simulink model "ChevilleNAO_Complete"  (R2015a)
settings: Solver=ode23t  StartTime=0.0  StopTime=2  MaxStep=0.001  RelTol=1e-3
undefined symbols (not defined in the file): X, Y, Z
libraries: sm_lib x306, fl_lib x13, nesl_utility x6
(part 1 of 7)
settings Model: CovSFcnEnable=off  Creator=Xavier  LastModifiedBy=Xavier
settings SolverCC: AlgebraicLoopSolver=LineSearch
settings DebuggingCC: SolverPrmCheckMsg=warning

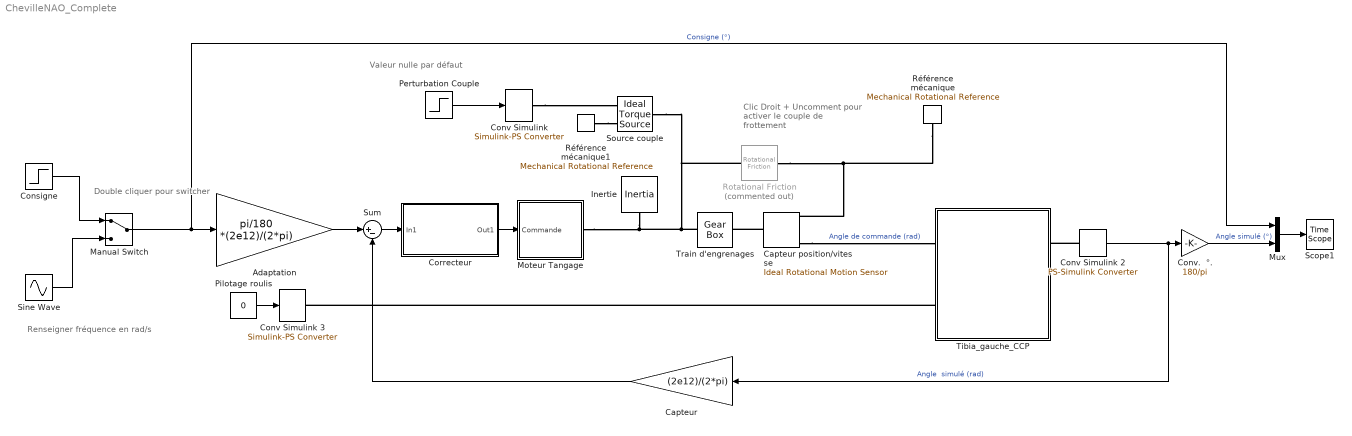
== system ChevilleNAO_Complete ==
  note: Clic Droit + Uncomment pour activer le couple de frottement
  note: Valeur nulle par défaut
  note: Double cliquer pour switcher
  note: Renseigner fréquence en rad/s
  Adaptation : Gain  Gain=pi/180 *(2e12)/(2*pi)
  Capteur : Gain  Gain=(2e12)/(2*pi)
  Capteur position/vitesse : fl_lib/Mechanical/Mechanical Sensors/Ideal Rotational Motion Sensor  offset=0 rad
  Consigne : Step  Time=0  After=5  SampleTime=0
  Conv Simulink 2 : nesl_utility/PS-Simulink Converter  PhysicalDomain=network_engine_domain  SubClassName=ps_output  LeftPortType=input  RightPortType=output  PseudoPeriodic=off  Frequencies=[]  Unit=1  AffineConversion=off
  Conv Simulink 3 : nesl_utility/Simulink-PS Converter  PhysicalDomain=network_engine_domain  SubClassName=ps_input  LeftPortType=input  RightPortType=output  PseudoPeriodic=off  Frequencies=[]  NoiseDistribution=none  NoiseParameters=[]  Unit=1  AffineConversion=off  InputFiltering=off  SimscapeFilterOrder=1  InputFilterTimeConstant=0.001  UdotUserProvided=1
  Conv Simulink : nesl_utility/Simulink-PS Converter  PhysicalDomain=network_engine_domain  SubClassName=ps_input  LeftPortType=input  RightPortType=output  PseudoPeriodic=off  Frequencies=[]  NoiseDistribution=none  NoiseParameters=[]  Unit=1  AffineConversion=off  InputFiltering=off  SimscapeFilterOrder=1  InputFilterTimeConstant=0.001  UdotUserProvided=1
  Conv.  °. : Gain  Gain=180/pi
  Correcteur : Subsystem
      mask Display: image(imread('carte.png'))
  Inertie : fl_lib/Mechanical/Rotational Elements/Inertia  inertia=4.8e-7 kg*m^2  w_specify=off  w_priority=High  w=0 rad/s  t_specify=off  t_priority=High  t=0 N*m
  Manual Switch : ManualSwitch
  Moteur Tangage : Subsystem
      mask Display: image(imread('moteur.png'))
  Mux : Mux  Inputs=2
  Perturbation Couple : Step  Time=0  After=-3.5E-3*0  SampleTime=0
  Pilotage roulis : Constant  Value=0
  Rotational Friction : fl_lib/Mechanical/Rotational Elements/Rotational Friction  Commented=on  brkwy_trq=5 mN*m  Col_trq=5 mN*m  visc_coef=10e-10 N*m/(rad/s)  trans_coef=10 s/rad  vel_thr=1e-4 rad/s  w_specify=off  w_priority=High  w=0 rad/s  t_specify=off  t_priority=High  t=0 N*m
  Référence mécanique : fl_lib/Mechanical/Rotational Elements/Mechanical Rotational Reference
  Référence mécanique1 : fl_lib/Mechanical/Rotational Elements/Mechanical Rotational Reference
  Scope1 : TimeScope
  Sine Wave : Sin  SampleTime=0
  Source couple : fl_lib/Mechanical/Mechanical Sources/Ideal Torque Source
  Sum : Sum  Inputs=|+-
  Tibia_gauche_CCP : Subsystem
      mask Display: image(imread('TibiaCCP.png'))
  Train d'engrenages : fl_lib/Mechanical/Mechanisms/Gear Box  ratio=130.85  t_in_specify=off  t_in_priority=High  t_in=0 N*m  t_out_specify=off  t_out_priority=High  t_out=0 N*m
  wires:
  Pilotage roulis/1 -> Conv Simulink 3/1
  Conv Simulink 2/1 -> Conv.  °./1, Capteur/1  "Angle  simulé (rad)"
  Manual Switch/1 -> Mux/1, Adaptation/1  "Consigne (°)"
  Adaptation/1 -> Sum/1
  Conv.  °./1 -> Mux/2  "Angle simulé (°)"
  Mux/1 -> Scope1/1
  Perturbation Couple/1 -> Conv Simulink/1
  Capteur/1 -> Sum/2
  Sum/1 -> Correcteur/1(In1)
  Correcteur/1(Out1) -> Moteur Tangage/1(Commande)
  Consigne/1 -> Manual Switch/1
  Sine Wave/1 -> Manual Switch/2
  connections:
  Train d'engrenages/LConn1 -- Rotational Friction/LConn1 -- Source couple/LConn1 -- Moteur Tangage/RConn1 -- Inertie/LConn1
  Tibia_gauche_CCP/LConn2 -- Conv Simulink 3/RConn1
  Capteur position/vitesse/LConn1 -- Train d'engrenages/RConn1
  Conv Simulink 2/LConn1 -- Tibia_gauche_CCP/RConn1
  Capteur position/vitesse/RConn3 -- Tibia_gauche_CCP/LConn1  "Angle de commande (rad)"
  Conv Simulink/RConn1 -- Source couple/RConn1
  Référence mécanique1/LConn1 -- Source couple/RConn2
  Référence mécanique/LConn1 -- Rotational Friction/RConn1 -- Capteur position/vitesse/RConn1

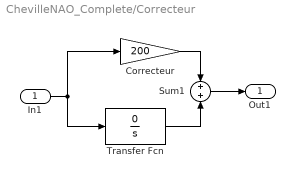
== system ChevilleNAO_Complete/Correcteur ==
  In1 : Inport
  Correcteur : Gain  Gain=200
  Sum1 : Sum
  Transfer Fcn : TransferFcn  Numerator=[0]  Denominator=[1 0]
  Out1 : Outport
  wires:
  In1/1 -> Transfer Fcn/1, Correcteur/1
  Sum1/1 -> Out1/1
  Transfer Fcn/1 -> Sum1/2
  Correcteur/1 -> Sum1/1

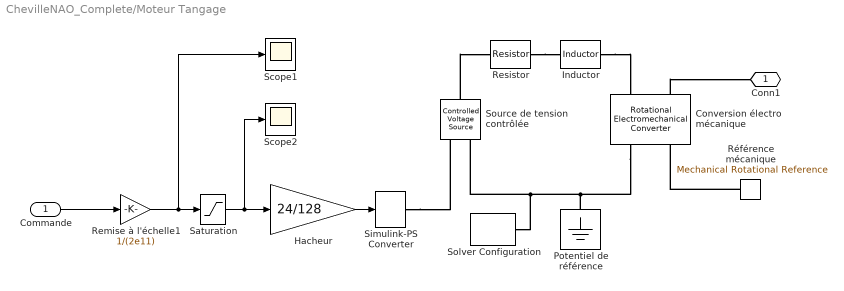
== system ChevilleNAO_Complete/Moteur Tangage ==
  Commande : Inport
  Conversion électro mécanique : fl_lib/Electrical/Electrical Elements/Rotational Electromechanical Converter  K=0.00203 V/rpm  i_specify=off  i_priority=High  i=0 A  v_specify=off  v_priority=High  v=0 V  t_specify=off  t_priority=High  t=0 N*m  w_specify=off  w_priority=High  w=0 rad/s
  Hacheur : Gain  Gain=24/128
  Inductor : fl_lib/Electrical/Electrical Elements/Inductor  l=0.6 mH  r=0 Ohm  g=1e-9 1/Ohm  i_specify=off  i_priority=High  i=0 A  v_specify=off  v_priority=High  v=0 V  i_L_specify=off  i_L_priority=High  i_L=0 A
  Potentiel de référence : fl_lib/Electrical/Electrical Elements/Electrical Reference
  Remise à l'échelle1 : Gain  Gain=1/(2e11)
  Resistor : fl_lib/Electrical/Electrical Elements/Resistor  R=5.4 Ohm  i_specify=off  i_priority=High  i=0 A  v_specify=off  v_priority=High  v=0 V
  Référence mécanique : fl_lib/Mechanical/Rotational Elements/Mechanical Rotational Reference
  Saturation : Saturate  UpperLimit=128  LowerLimit=-128
  Scope1 : Scope
      settings: TimeRange=0.7  YMin=0  YMax=70
  Scope2 : Scope
      settings: TimeRange=1  YMin=0  YMax=60  SaveName=ScopeData3
  Simulink-PS Converter : nesl_utility/Simulink-PS Converter  PhysicalDomain=network_engine_domain  SubClassName=ps_input  LeftPortType=input  RightPortType=output  PseudoPeriodic=off  Frequencies=[]  NoiseDistribution=none  NoiseParameters=[]  Unit=1  AffineConversion=off  InputFiltering=off  SimscapeFilterOrder=1  InputFilterTimeConstant=0.001  UdotUserProvided=1
  Solver Configuration : nesl_utility/Solver Configuration  PhysicalDomain=network_engine_domain  SubClassName=solver  LeftPortType=input  RightPortType=generic  Accelerate=off  Tones=[]  Harmonics=[]  SimulateNoise=off  Profile=off  UseLocalSampling=off  EnableSwitchedLinearOptims=on  FrequencyDomain=off  UseCCode=off  RelTol=0.001  AbsTol=1e-06  MinStep=1e-09  ToWorkspace=off  RevertToSquareIcSolve=off  NumHomotopyIterations=100  DoDC=off  ResidualTolerance=1e-09  UseLocalSolver=off  LocalSolverChoice=NE_BACKWARD_EULER_ADVANCER  LocalSolverSampleTime=0.001  DoFixedCost=off  MaxNonlinIter=3  MaxModeIter=2  LinearAlgebra=Sparse  DelaysMemoryBudget=1024  AutomaticFiltering=on  FilteringTimeConstant=0.001
  Source de tension contrôlée : fl_lib/Electrical/Electrical Sources/Controlled Voltage Source
  Conn1 : PMIOPort  Port=1  Side=Right
  wires:
  Saturation/1 -> Scope2/1, Hacheur/1
  Hacheur/1 -> Simulink-PS Converter/1
  Commande/1 -> Remise à l'échelle1/1
  Remise à l'échelle1/1 -> Scope1/1, Saturation/1
  connections:
  Conversion électro mécanique/LConn2 -- Conn1/RConn1
  Référence mécanique/LConn1 -- Conversion électro mécanique/RConn2
  Source de tension contrôlée/LConn1 -- Resistor/LConn1
  Resistor/RConn1 -- Inductor/LConn1
  Inductor/RConn1 -- Conversion électro mécanique/LConn1
  Conversion électro mécanique/RConn1 -- Potentiel de référence/LConn1 -- Solver Configuration/RConn1 -- Source de tension contrôlée/RConn2
  Simulink-PS Converter/RConn1 -- Source de tension contrôlée/RConn1

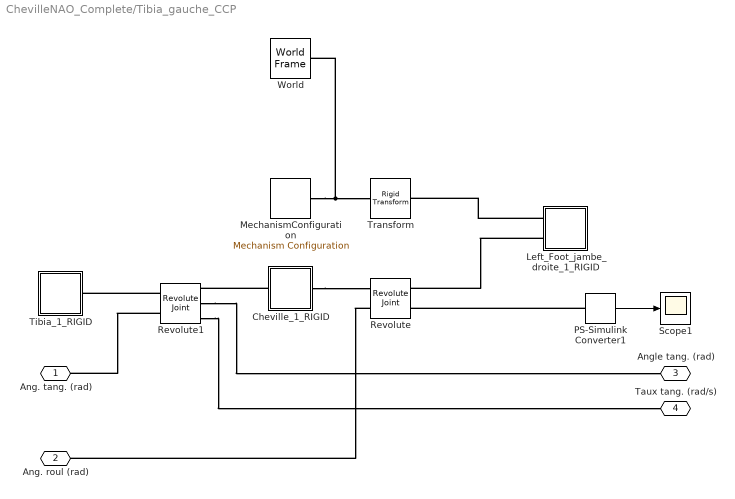
== system ChevilleNAO_Complete/Tibia_gauche_CCP ==
  Cheville_1_RIGID : Subsystem
  Left_Foot_jambe_droite_1_RIGID : Subsystem
  MechanismConfiguration : sm_lib/Utilities/Mechanism Configuration  UniformGravity=Constant  GravityVector=[0 -9.81 0]  GravityUnits=m/s^2  LinearizationDelta=0.001  BlockFunction=simmechanics.library.utilities.mechanism_configuration
  PS-Simulink Converter1 : nesl_utility/PS-Simulink Converter  PhysicalDomain=network_engine_domain  SubClassName=ps_output  LeftPortType=input  RightPortType=output  PseudoPeriodic=off  Frequencies=[]  Unit=1  AffineConversion=off
  Revolute : sm_lib/Joints/Revolute Joint  SenseConstraintForce=off  SenseConstraintForceX=off  SenseConstraintForceY=off  SenseConstraintForceZ=off  SenseConstraintTorque=off  SenseConstraintTorqueX=off  SenseConstraintTorqueY=off  SenseConstraintTorqueZ=off  SenseTotalForce=off  SenseTotalForceX=off  SenseTotalForceY=off  SenseTotalForceZ=off  SenseTotalTorque=off  SenseTotalTorqueX=off  SenseTotalTorqueY=off  SenseTotalTorqueZ=off  CompositeWrenchDir=FollowerOnBase  CompositeWrenchFrame=BaseFrame  EquilibriumPosition=0  EquilibriumPositionUnits=rad  SpringStiffness=0  SpringStiffnessUnits=m*N/rad  DampingCoefficient=0  DampingCoefficientUnits=m*s*N/rad  TorqueActuationMode=ComputedTorque  MotionActuationMode=InputMotion  SensePosition=on  SenseVelocity=off  SenseAcceleration=off  SenseTorqueForce=off  PositionTargetSpecify=off  PositionTargetPriority=Low  PositionTargetValue=-1.5107634736951701e-14  PositionTargetValueUnits=deg  VelocityTargetSpecify=off  VelocityTargetPriority=High  VelocityTargetValue=0  VelocityTargetValueUnits=deg/s  BlockFunction=simmechanics.library.joints.revolute_joint
  Revolute1 : sm_lib/Joints/Revolute Joint  SenseConstraintForce=off  SenseConstraintForceX=off  SenseConstraintForceY=off  SenseConstraintForceZ=off  SenseConstraintTorque=off  SenseConstraintTorqueX=off  SenseConstraintTorqueY=off  SenseConstraintTorqueZ=off  SenseTotalForce=off  SenseTotalForceX=off  SenseTotalForceY=off  SenseTotalForceZ=off  SenseTotalTorque=off  SenseTotalTorqueX=off  SenseTotalTorqueY=off  SenseTotalTorqueZ=off  CompositeWrenchDir=FollowerOnBase  CompositeWrenchFrame=BaseFrame  EquilibriumPosition=0  EquilibriumPositionUnits=rad  SpringStiffness=0  SpringStiffnessUnits=m*N/rad  DampingCoefficient=0  DampingCoefficientUnits=m*s*N/rad  TorqueActuationMode=ComputedTorque  MotionActuationMode=InputMotion  SensePosition=on  SenseVelocity=on  SenseAcceleration=off  SenseTorqueForce=off  PositionTargetSpecify=on  PositionTargetPriority=Low  PositionTargetValue=-110  PositionTargetValueUnits=deg  VelocityTargetSpecify=off  VelocityTargetPriority=High  VelocityTargetValue=0  VelocityTargetValueUnits=deg/s  BlockFunction=simmechanics.library.joints.revolute_joint
  Scope1 : Scope
      settings: TimeRange=1  YMin=0  YMax=60  SaveName=ScopeData2
  Tibia_1_RIGID : Subsystem
  Transform : sm_lib/Frames and Transforms/Rigid Transform  TranslationMethod=Cartesian  TranslationLengthUnit=mm  TranslationStandardAxis=+Z  TranslationStandardOffset=0  TranslationCartesianOffset=[-0.025653108819686382 -0.048676846529821009 -0.10751598813965911]  TranslationROffset=0  TranslationROffsetUnits=m  TranslationZOffset=0  TranslationZOffsetUnits=m  TranslationThetaOffset=0  TranslationThetaOffsetUnits=deg  RotationMethod=ArbitraryAxis  RotationAngleUnits=rad  RotationStandardAxis=+Z  RotationAngle=1.5707963267948961  RotationArbitraryAxis=[-1.3877787807814457e-16 -1 -1.5265566588595902e-16]  FollAlignAxisA=+X  BaseAlignAxisA=+Y  FollAlignAxisB=+Y  BaseAlignAxisB=+Z  RotationMatrix=[1 0 0; 0 1 0; 0 0 1]  BlockFunction=simmechanics.library.frames_transforms.rigid_transform
  World : sm_lib/Frames and Transforms/World Frame  BlockFunction=simmechanics.library.frames_transforms.world_frame
  Ang. tang. (rad) : PMIOPort  Port=1  Side=Left
  Ang. roul (rad) : PMIOPort  Port=2  Side=Left
  Angle tang. (rad) : PMIOPort  Port=3  Side=Right
  Taux tang. (rad/s) : PMIOPort  Port=4  Side=Right
  wires:
  PS-Simulink Converter1/1 -> Scope1/1
  connections:
  World/RConn1 -- Transform/LConn1 -- MechanismConfiguration/RConn1
  Cheville_1_RIGID/RConn1 -- Revolute/LConn1
  Left_Foot_jambe_droite_1_RIGID/LConn2 -- Revolute/RConn1
  Revolute1/LConn1 -- Tibia_1_RIGID/RConn1
  Cheville_1_RIGID/LConn1 -- Revolute1/RConn1
  Left_Foot_jambe_droite_1_RIGID/LConn1 -- Transform/RConn1
  Revolute1/LConn2 -- Ang. tang. (rad)/RConn1
  Revolute/LConn2 -- Ang. roul (rad)/RConn1
  Revolute1/RConn2 -- Angle tang. (rad)/RConn1
  PS-Simulink Converter1/LConn1 -- Revolute/RConn2
  Revolute1/RConn3 -- Taux tang. (rad/s)/RConn1

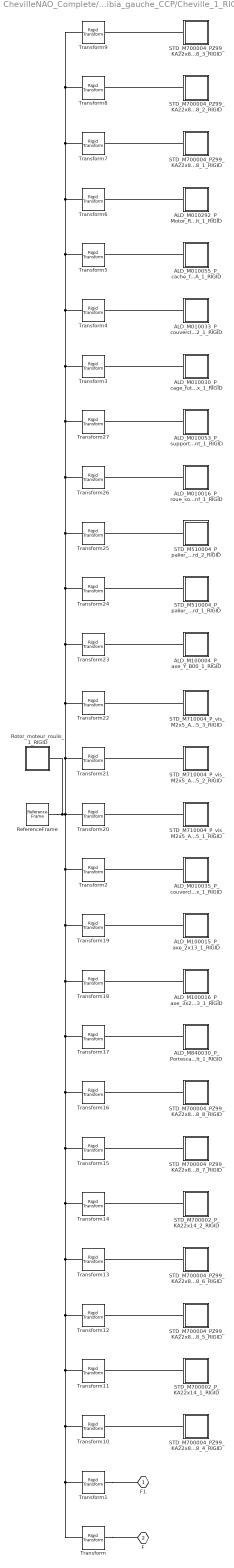
== system ChevilleNAO_Complete/Tibia_gauche_CCP/Cheville_1_RIGID ==
  ALD_M010016_P_roue_sortie_inf_1_RIGID : Subsystem
  ALD_M010030_P_cage_fut_moteur_cheville_gauche_Axx_1_RIGID : Subsystem
  ALD_M010033_P_couvercle_X_AV_cheville_A02_1_RIGID : Subsystem
  ALD_M010035_P_couvercle_X_AR_Axx_1_RIGID : Subsystem
  ALD_M010053_P_support_aimant_1_RIGID : Subsystem
  ALD_M010055_P_cache_fut_moteur_cheville_A_1_RIGID : Subsystem
  ALD_M010292_P_Motor_Ring_Default_1_RIGID : Subsystem
  ALD_M100004_P_axe_Y_B00_1_RIGID : Subsystem
  ALD_M100015_P_axe_2x13_1_RIGID : Subsystem
  ALD_M100016_P_axe_3x27_3_1_RIGID : Subsystem
  ALD_M840030_P_Portescap_22NT_82_213P_Z13_Default_1_RIGID : Subsystem
  ReferenceFrame : sm_lib/Frames and Transforms/Reference Frame  BlockFunction=simmechanics.library.frames_transforms.reference_frame
  Rotor_moteur_roulis_1_RIGID : Subsystem
  STD_M510004_P_palier_GFM_1517_05_stabdard_1_RIGID : Subsystem
  STD_M510004_P_palier_GFM_1517_05_stabdard_2_RIGID : Subsystem
  STD_M700002_P_KA22x14_1_RIGID : Subsystem
  STD_M700002_P_KA22x14_2_RIGID : Subsystem
  STD_M700004_PZ99_KA22x8_KA22_x_8_1_RIGID : Subsystem
  STD_M700004_PZ99_KA22x8_KA22_x_8_2_RIGID : Subsystem
  STD_M700004_PZ99_KA22x8_KA22_x_8_3_RIGID : Subsystem
  STD_M700004_PZ99_KA22x8_KA22_x_8_4_RIGID : Subsystem
  STD_M700004_PZ99_KA22x8_KA22_x_8_5_RIGID : Subsystem
  STD_M700004_PZ99_KA22x8_KA22_x_8_6_RIGID : Subsystem
  STD_M700004_PZ99_KA22x8_KA22_x_8_7_RIGID : Subsystem
  STD_M700004_PZ99_KA22x8_KA22_x_8_8_RIGID : Subsystem
  STD_M710004_P_vis_M2x5_ALD_M710004_PZ99_vis_M2x5_1_RIGID : Subsystem
  STD_M710004_P_vis_M2x5_ALD_M710004_PZ99_vis_M2x5_2_RIGID : Subsystem
  STD_M710004_P_vis_M2x5_ALD_M710004_PZ99_vis_M2x5_3_RIGID : Subsystem
  Transform : sm_lib/Frames and Transforms/Rigid Transform  TranslationMethod=Cartesian  TranslationLengthUnit=mm  TranslationStandardAxis=+Z  TranslationStandardOffset=0  TranslationCartesianOffset=[-7.1054273576010019e-15 -2.699999999999994 106.70000000000005]  TranslationROffset=0  TranslationROffsetUnits=m  TranslationZOffset=0  TranslationZOffsetUnits=m  TranslationThetaOffset=0  TranslationThetaOffsetUnits=deg  RotationMethod=ArbitraryAxis  RotationAngleUnits=rad  RotationStandardAxis=+Z  RotationAngle=3.1415926535897931  RotationArbitraryAxis=[-1 1.3684555315672042e-48 -1.1102230246251565e-16]  FollAlignAxisA=+X  BaseAlignAxisA=+Y  FollAlignAxisB=+Y  BaseAlignAxisB=+Z  RotationMatrix=[1 0 0; 0 1 0; 0 0 1]  BlockFunction=simmechanics.library.frames_transforms.rigid_transform
  Transform1 : sm_lib/Frames and Transforms/Rigid Transform  TranslationMethod=Cartesian  TranslationLengthUnit=mm  TranslationStandardAxis=+Z  TranslationStandardOffset=0  TranslationCartesianOffset=[19.100000000000037 -2.6999999999999695 69.300000000000097]  TranslationROffset=0  TranslationROffsetUnits=m  TranslationZOffset=0  TranslationZOffsetUnits=m  TranslationThetaOffset=0  TranslationThetaOffsetUnits=deg  RotationMethod=ArbitraryAxis  RotationAngleUnits=rad  RotationStandardAxis=+Z  RotationAngle=2.0943951023931953  RotationArbitraryAxis=[-0.57735026918962562 -0.57735026918962584 0.57735026918962595]  FollAlignAxisA=+X  BaseAlignAxisA=+Y  FollAlignAxisB=+Y  BaseAlignAxisB=+Z  RotationMatrix=[1 0 0; 0 1 0; 0 0 1]  BlockFunction=simmechanics.library.frames_transforms.rigid_transform
  Transform10 : sm_lib/Frames and Transforms/Rigid Transform  TranslationMethod=Cartesian  TranslationLengthUnit=mm  TranslationStandardAxis=+Z  TranslationStandardOffset=0  TranslationCartesianOffset=[-11.350000000000009 -11.200000000000015 98.900000000000063]  TranslationROffset=0  TranslationROffsetUnits=m  TranslationZOffset=0  TranslationZOffsetUnits=m  TranslationThetaOffset=0  TranslationThetaOffsetUnits=deg  RotationMethod=ArbitraryAxis  RotationAngleUnits=rad  RotationStandardAxis=+Z  RotationAngle=1.9006984205029975  RotationArbitraryAxis=[-0.49465614020694099 0.71458421890715063 0.49465614020694076]  FollAlignAxisA=+X  BaseAlignAxisA=+Y  FollAlignAxisB=+Y  BaseAlignAxisB=+Z  RotationMatrix=[1 0 0; 0 1 0; 0 0 1]  BlockFunction=simmechanics.library.frames_transforms.rigid_transform
  Transform11 : sm_lib/Frames and Transforms/Rigid Transform  TranslationMethod=Cartesian  TranslationLengthUnit=mm  TranslationStandardAxis=+Z  TranslationStandardOffset=0  TranslationCartesianOffset=[11.099999999999984 8.9612955438671822 30.200000000007652]  TranslationROffset=0  TranslationROffsetUnits=m  TranslationZOffset=0  TranslationZOffsetUnits=m  TranslationThetaOffset=0  TranslationThetaOffsetUnits=deg  RotationMethod=ArbitraryAxis  RotationAngleUnits=rad  RotationStandardAxis=+Z  RotationAngle=1.5707963267948968  RotationArbitraryAxis=[1.8986906709276627e-16 -1 1.8986906709276627e-16]  FollAlignAxisA=+X  BaseAlignAxisA=+Y  FollAlignAxisB=+Y  BaseAlignAxisB=+Z  RotationMatrix=[1 0 0; 0 1 0; 0 0 1]  BlockFunction=simmechanics.library.frames_transforms.rigid_transform
  Transform12 : sm_lib/Frames and Transforms/Rigid Transform  TranslationMethod=Cartesian  TranslationLengthUnit=mm  TranslationStandardAxis=+Z  TranslationStandardOffset=0  TranslationCartesianOffset=[11.349999999999987 -11.19999999999999 34.700000000000038]  TranslationROffset=0  TranslationROffsetUnits=m  TranslationZOffset=0  TranslationZOffsetUnits=m  TranslationThetaOffset=0  TranslationThetaOffsetUnits=deg  RotationMethod=ArbitraryAxis  RotationAngleUnits=rad  RotationStandardAxis=+Z  RotationAngle=2.4847534573610446  RotationArbitraryAxis=[0.66478666552019172 -0.34076000160389858 0.66478666552019205]  FollAlignAxisA=+X  BaseAlignAxisA=+Y  FollAlignAxisB=+Y  BaseAlignAxisB=+Z  RotationMatrix=[1 0 0; 0 1 0; 0 0 1]  BlockFunction=simmechanics.library.frames_transforms.rigid_transform
  Transform13 : sm_lib/Frames and Transforms/Rigid Transform  TranslationMethod=Cartesian  TranslationLengthUnit=mm  TranslationStandardAxis=+Z  TranslationStandardOffset=0  TranslationCartesianOffset=[-11.35000000000001 -11.19999999999999 34.700000000000024]  TranslationROffset=0  TranslationROffsetUnits=m  TranslationZOffset=0  TranslationZOffsetUnits=m  TranslationThetaOffset=0  TranslationThetaOffsetUnits=deg  RotationMethod=ArbitraryAxis  RotationAngleUnits=rad  RotationStandardAxis=+Z  RotationAngle=3.0141447602302587  RotationArbitraryAxis=[-0.70566572829829377 -0.063810342503989731 -0.70566572829829421]  FollAlignAxisA=+X  BaseAlignAxisA=+Y  FollAlignAxisB=+Y  BaseAlignAxisB=+Z  RotationMatrix=[1 0 0; 0 1 0; 0 0 1]  BlockFunction=simmechanics.library.frames_transforms.rigid_transform
  Transform14 : sm_lib/Frames and Transforms/Rigid Transform  TranslationMethod=Cartesian  TranslationLengthUnit=mm  TranslationStandardAxis=+Z  TranslationStandardOffset=0  TranslationCartesianOffset=[-11.1 8.9612955438669868 30.20000000000767]  TranslationROffset=0  TranslationROffsetUnits=m  TranslationZOffset=0  TranslationZOffsetUnits=m  TranslationThetaOffset=0  TranslationThetaOffsetUnits=deg  RotationMethod=ArbitraryAxis  RotationAngleUnits=rad  RotationStandardAxis=+Z  RotationAngle=3.0743876947638533  RotationArbitraryAxis=[-0.70670716102281805 -0.033615132279040408 -0.70670716102281805]  FollAlignAxisA=+X  BaseAlignAxisA=+Y  FollAlignAxisB=+Y  BaseAlignAxisB=+Z  RotationMatrix=[1 0 0; 0 1 0; 0 0 1]  BlockFunction=simmechanics.library.frames_transforms.rigid_transform
  Transform15 : sm_lib/Frames and Transforms/Rigid Transform  TranslationMethod=Cartesian  TranslationLengthUnit=mm  TranslationStandardAxis=+Z  TranslationStandardOffset=0  TranslationCartesianOffset=[0 -14.19999999999999 34.70000000000001]  TranslationROffset=0  TranslationROffsetUnits=m  TranslationZOffset=0  TranslationZOffsetUnits=m  TranslationThetaOffset=0  TranslationThetaOffsetUnits=deg  RotationMethod=ArbitraryAxis  RotationAngleUnits=rad  RotationStandardAxis=+Z  RotationAngle=2.8742390574163252  RotationArbitraryAxis=[0.70068375846550734 -0.13447877618903373 0.7006837584655079]  FollAlignAxisA=+X  BaseAlignAxisA=+Y  FollAlignAxisB=+Y  BaseAlignAxisB=+Z  RotationMatrix=[1 0 0; 0 1 0; 0 0 1]  BlockFunction=simmechanics.library.frames_transforms.rigid_transform
  Transform16 : sm_lib/Frames and Transforms/Rigid Transform  TranslationMethod=Cartesian  TranslationLengthUnit=mm  TranslationStandardAxis=+Z  TranslationStandardOffset=0  TranslationCartesianOffset=[-11.350000000000033 24.799999999999994 98.900000000000077]  TranslationROffset=0  TranslationROffsetUnits=m  TranslationZOffset=0  TranslationZOffsetUnits=m  TranslationThetaOffset=0  TranslationThetaOffsetUnits=deg  RotationMethod=ArbitraryAxis  RotationAngleUnits=rad  RotationStandardAxis=+Z  RotationAngle=1.6880721668474532  RotationArbitraryAxis=[0.32365200516053011 0.88909997138181041 -0.32365200516053033]  FollAlignAxisA=+X  BaseAlignAxisA=+Y  FollAlignAxisB=+Y  BaseAlignAxisB=+Z  RotationMatrix=[1 0 0; 0 1 0; 0 0 1]  BlockFunction=simmechanics.library.frames_transforms.rigid_transform
  Transform17 : sm_lib/Frames and Transforms/Rigid Transform  TranslationMethod=Cartesian  TranslationLengthUnit=mm  TranslationStandardAxis=+Z  TranslationStandardOffset=0  TranslationCartesianOffset=[0 -0.59999999999999121 54.041022897086762]  TranslationROffset=0  TranslationROffsetUnits=m  TranslationZOffset=0  TranslationZOffsetUnits=m  TranslationThetaOffset=0  TranslationThetaOffsetUnits=deg  RotationMethod=ArbitraryAxis  RotationAngleUnits=rad  RotationStandardAxis=+Z  RotationAngle=2.8342931083834251  RotationArbitraryAxis=[0.15487043520039936 -0.69857538902427663 -0.69857538902427663]  FollAlignAxisA=+X  BaseAlignAxisA=+Y  FollAlignAxisB=+Y  BaseAlignAxisB=+Z  RotationMatrix=[1 0 0; 0 1 0; 0 0 1]  BlockFunction=simmechanics.library.frames_transforms.rigid_transform
  Transform18 : sm_lib/Frames and Transforms/Rigid Transform  TranslationMethod=Cartesian  TranslationLengthUnit=mm  TranslationStandardAxis=+Z  TranslationStandardOffset=0  TranslationCartesianOffset=[0 13.80000000000001 108.25000000000004]  TranslationROffset=0  TranslationROffsetUnits=m  TranslationZOffset=0  TranslationZOffsetUnits=m  TranslationThetaOffset=0  TranslationThetaOffsetUnits=deg  RotationMethod=ArbitraryAxis  RotationAngleUnits=rad  RotationStandardAxis=+Z  RotationAngle=3.1415926535897931  RotationArbitraryAxis=[0.99350698871525212 0.11377110078553444 0]  FollAlignAxisA=+X  BaseAlignAxisA=+Y  FollAlignAxisB=+Y  BaseAlignAxisB=+Z  RotationMatrix=[1 0 0; 0 1 0; 0 0 1]  BlockFunction=simmechanics.library.frames_transforms.rigid_transform
  Transform19 : sm_lib/Frames and Transforms/Rigid Transform  TranslationMethod=Cartesian  TranslationLengthUnit=mm  TranslationStandardAxis=+Z  TranslationStandardOffset=0  TranslationCartesianOffset=[0 -0.59999999999998943 100.10000000000002]  TranslationROffset=0  TranslationROffsetUnits=m  TranslationZOffset=0  TranslationZOffsetUnits=m  TranslationThetaOffset=0  TranslationThetaOffsetUnits=deg  RotationMethod=ArbitraryAxis  RotationAngleUnits=rad  RotationStandardAxis=+Z  RotationAngle=3.1415926535897931  RotationArbitraryAxis=[-0.60689117566578277 0.79478494003032296 -2.787447066723693e-16]  FollAlignAxisA=+X  BaseAlignAxisA=+Y  FollAlignAxisB=+Y  BaseAlignAxisB=+Z  RotationMatrix=[1 0 0; 0 1 0; 0 0 1]  BlockFunction=simmechanics.library.frames_transforms.rigid_transform
  Transform2 : sm_lib/Frames and Transforms/Rigid Transform  TranslationMethod=Cartesian  TranslationLengthUnit=mm  TranslationStandardAxis=+Z  TranslationStandardOffset=0  TranslationCartesianOffset=[0 0 42.700000000000031]  TranslationROffset=0  TranslationROffsetUnits=m  TranslationZOffset=0  TranslationZOffsetUnits=m  TranslationThetaOffset=0  TranslationThetaOffsetUnits=deg  RotationMethod=ArbitraryAxis  RotationAngleUnits=rad  RotationStandardAxis=+Z  RotationAngle=3.1415926535897931  RotationArbitraryAxis=[-5.5511151231257852e-17 1 0]  FollAlignAxisA=+X  BaseAlignAxisA=+Y  FollAlignAxisB=+Y  BaseAlignAxisB=+Z  RotationMatrix=[1 0 0; 0 1 0; 0 0 1]  BlockFunction=simmechanics.library.frames_transforms.rigid_transform
  Transform20 : sm_lib/Frames and Transforms/Rigid Transform  TranslationMethod=Cartesian  TranslationLengthUnit=mm  TranslationStandardAxis=+Z  TranslationStandardOffset=0  TranslationCartesianOffset=[4.9149122657339559 -3.4414586181062545 83.900000000000034]  TranslationROffset=0  TranslationROffsetUnits=m  TranslationZOffset=0  TranslationZOffsetUnits=m  TranslationThetaOffset=0  TranslationThetaOffsetUnits=deg  RotationMethod=ArbitraryAxis  RotationAngleUnits=rad  RotationStandardAxis=+Z  RotationAngle=2.7095537269323366  RotationArbitraryAxis=[-0.68987119699943567 0.21944353055201188 0.68987119699943567]  FollAlignAxisA=+X  BaseAlignAxisA=+Y  FollAlignAxisB=+Y  BaseAlignAxisB=+Z  RotationMatrix=[1 0 0; 0 1 0; 0 0 1]  BlockFunction=simmechanics.library.frames_transforms.rigid_transform
  Transform21 : sm_lib/Frames and Transforms/Rigid Transform  TranslationMethod=Cartesian  TranslationLengthUnit=mm  TranslationStandardAxis=+Z  TranslationStandardOffset=0  TranslationCartesianOffset=[-4.9149122657339674 3.441458618106283 83.900000000000034]  TranslationROffset=0  TranslationROffsetUnits=m  TranslationZOffset=0  TranslationZOffsetUnits=m  TranslationThetaOffset=0  TranslationThetaOffsetUnits=deg  RotationMethod=ArbitraryAxis  RotationAngleUnits=rad  RotationStandardAxis=+Z  RotationAngle=3.0385834060669552  RotationArbitraryAxis=[-0.70616661467566355 0.051550214694275308 0.70616661467566355]  FollAlignAxisA=+X  BaseAlignAxisA=+Y  FollAlignAxisB=+Y  BaseAlignAxisB=+Z  RotationMatrix=[1 0 0; 0 1 0; 0 0 1]  BlockFunction=simmechanics.library.frames_transforms.rigid_transform
  Transform22 : sm_lib/Frames and Transforms/Rigid Transform  TranslationMethod=Cartesian  TranslationLengthUnit=mm  TranslationStandardAxis=+Z  TranslationStandardOffset=0  TranslationCartesianOffset=[5.4378467222198914 2.5357095704442316 83.900000000000034]  TranslationROffset=0  TranslationROffsetUnits=m  TranslationZOffset=0  TranslationZOffsetUnits=m  TranslationThetaOffset=0  TranslationThetaOffsetUnits=deg  RotationMethod=ArbitraryAxis  RotationAngleUnits=rad  RotationStandardAxis=+Z  RotationAngle=1.571360462234191  RotationArbitraryAxis=[0.023744838176873326 0.99943602362527839 -0.023744838176873326]  FollAlignAxisA=+X  BaseAlignAxisA=+Y  FollAlignAxisB=+Y  BaseAlignAxisB=+Z  RotationMatrix=[1 0 0; 0 1 0; 0 0 1]  BlockFunction=simmechanics.library.frames_transforms.rigid_transform
  Transform23 : sm_lib/Frames and Transforms/Rigid Transform  TranslationMethod=Cartesian  TranslationLengthUnit=mm  TranslationStandardAxis=+Z  TranslationStandardOffset=0  TranslationCartesianOffset=[-15.400000000000036 -2.699999999999994 69.300000000000026]  TranslationROffset=0  TranslationROffsetUnits=m  TranslationZOffset=0  TranslationZOffsetUnits=m  TranslationThetaOffset=0  TranslationThetaOffsetUnits=deg  RotationMethod=ArbitraryAxis  RotationAngleUnits=rad  RotationStandardAxis=+Z  RotationAngle=3.119204624685064  RotationArbitraryAxis=[-0.70706247375036735 0.70706247375036502 0.011194482034708355]  FollAlignAxisA=+X  BaseAlignAxisA=+Y  FollAlignAxisB=+Y  BaseAlignAxisB=+Z  RotationMatrix=[1 0 0; 0 1 0; 0 0 1]  BlockFunction=simmechanics.library.frames_transforms.rigid_transform
  Transform24 : sm_lib/Frames and Transforms/Rigid Transform  TranslationMethod=Cartesian  TranslationLengthUnit=mm  TranslationStandardAxis=+Z  TranslationStandardOffset=0  TranslationCartesianOffset=[14.300000000000034 -2.7000000000000495 69.300000000000125]  TranslationROffset=0  TranslationROffsetUnits=m  TranslationZOffset=0  TranslationZOffsetUnits=m  TranslationThetaOffset=0  TranslationThetaOffsetUnits=deg  RotationMethod=ArbitraryAxis  RotationAngleUnits=rad  RotationStandardAxis=+Z  RotationAngle=1.0009709594344269  RotationArbitraryAxis=[1 0 0]  FollAlignAxisA=+X  BaseAlignAxisA=+Y  FollAlignAxisB=+Y  BaseAlignAxisB=+Z  RotationMatrix=[1 0 0; 0 1 0; 0 0 1]  BlockFunction=simmechanics.library.frames_transforms.rigid_transform
  Transform25 : sm_lib/Frames and Transforms/Rigid Transform  TranslationMethod=Cartesian  TranslationLengthUnit=mm  TranslationStandardAxis=+Z  TranslationStandardOffset=0  TranslationCartesianOffset=[-14.300000000000043 -2.700000000000244 69.300000000000054]  TranslationROffset=0  TranslationROffsetUnits=m  TranslationZOffset=0  TranslationZOffsetUnits=m  TranslationThetaOffset=0  TranslationThetaOffsetUnits=deg  RotationMethod=ArbitraryAxis  RotationAngleUnits=rad  RotationStandardAxis=+Z  RotationAngle=3.1415926535897931  RotationArbitraryAxis=[0 0.96684798613633138 -0.25535264185850998]  FollAlignAxisA=+X  BaseAlignAxisA=+Y  FollAlignAxisB=+Y  BaseAlignAxisB=+Z  RotationMatrix=[1 0 0; 0 1 0; 0 0 1]  BlockFunction=simmechanics.library.frames_transforms.rigid_transform
  Transform26 : sm_lib/Frames and Transforms/Rigid Transform  TranslationMethod=Cartesian  TranslationLengthUnit=mm  TranslationStandardAxis=+Z  TranslationStandardOffset=0  TranslationCartesianOffset=[-19.900000000000457 -2.6999999999999802 69.300000000000111]  TranslationROffset=0  TranslationROffsetUnits=m  TranslationZOffset=0  TranslationZOffsetUnits=m  TranslationThetaOffset=0  TranslationThetaOffsetUnits=deg  RotationMethod=ArbitraryAxis  RotationAngleUnits=rad  RotationStandardAxis=+Z  RotationAngle=1.7177715174584005  RotationArbitraryAxis=[0.35740674433659209 -0.35740674433659209 0.86285620946101771]  FollAlignAxisA=+X  BaseAlignAxisA=+Y  FollAlignAxisB=+Y  BaseAlignAxisB=+Z  RotationMatrix=[1 0 0; 0 1 0; 0 0 1]  BlockFunction=simmechanics.library.frames_transforms.rigid_transform
  Transform27 : sm_lib/Frames and Transforms/Rigid Transform  TranslationMethod=Cartesian  TranslationLengthUnit=mm  TranslationStandardAxis=+Z  TranslationStandardOffset=0  TranslationCartesianOffset=[0 -2.700000000000105 100.80000000000008]  TranslationROffset=0  TranslationROffsetUnits=m  TranslationZOffset=0  TranslationZOffsetUnits=m  TranslationThetaOffset=0  TranslationThetaOffsetUnits=deg  RotationMethod=ArbitraryAxis  RotationAngleUnits=rad  RotationStandardAxis=+Z  RotationAngle=2.4188584057763838  RotationArbitraryAxis=[0.37796447300922598 -0.65465367070797675 -0.6546536707079782]  FollAlignAxisA=+X  BaseAlignAxisA=+Y  FollAlignAxisB=+Y  BaseAlignAxisB=+Z  RotationMatrix=[1 0 0; 0 1 0; 0 0 1]  BlockFunction=simmechanics.library.frames_transforms.rigid_transform
  Transform3 : sm_lib/Frames and Transforms/Rigid Transform  TranslationMethod=None  TranslationLengthUnit=m  TranslationStandardAxis=+Z  TranslationStandardOffset=0  TranslationCartesianOffset=[0 0 0]  TranslationROffset=0  TranslationROffsetUnits=m  TranslationZOffset=0  TranslationZOffsetUnits=m  TranslationThetaOffset=0  TranslationThetaOffsetUnits=deg  RotationMethod=None  RotationAngleUnits=deg  RotationStandardAxis=+Z  RotationAngle=0.0  RotationArbitraryAxis=[0 0 1]  FollAlignAxisA=+X  BaseAlignAxisA=+Y  FollAlignAxisB=+Y  BaseAlignAxisB=+Z  RotationMatrix=[1 0 0; 0 1 0; 0 0 1]  BlockFunction=simmechanics.library.frames_transforms.rigid_transform
  Transform4 : sm_lib/Frames and Transforms/Rigid Transform  TranslationMethod=Cartesian  TranslationLengthUnit=mm  TranslationStandardAxis=+Z  TranslationStandardOffset=0  TranslationCartesianOffset=[-14.100000000000005 0 81.000000000000043]  TranslationROffset=0  TranslationROffsetUnits=m  TranslationZOffset=0  TranslationZOffsetUnits=m  TranslationThetaOffset=0  TranslationThetaOffsetUnits=deg  RotationMethod=ArbitraryAxis  RotationAngleUnits=rad  RotationStandardAxis=+Z  RotationAngle=1.5707963267948968  RotationArbitraryAxis=[1.9428902930940235e-16 -1 1.9428902930940235e-16]  FollAlignAxisA=+X  BaseAlignAxisA=+Y  FollAlignAxisB=+Y  BaseAlignAxisB=+Z  RotationMatrix=[1 0 0; 0 1 0; 0 0 1]  BlockFunction=simmechanics.library.frames_transforms.rigid_transform
  Transform5 : sm_lib/Frames and Transforms/Rigid Transform  TranslationMethod=Cartesian  TranslationLengthUnit=mm  TranslationStandardAxis=+Z  TranslationStandardOffset=0  TranslationCartesianOffset=[14.100000000006899 -1.2101430968414206e-11 -1.0755285551056204e-10]  TranslationROffset=0  TranslationROffsetUnits=m  TranslationZOffset=0  TranslationZOffsetUnits=m  TranslationThetaOffset=0  TranslationThetaOffsetUnits=deg  RotationMethod=ArbitraryAxis  RotationAngleUnits=rad  RotationStandardAxis=+Z  RotationAngle=1.5707963267948968  RotationArbitraryAxis=[-6.2450045135165228e-17 1 2.1510571102112373e-16]  FollAlignAxisA=+X  BaseAlignAxisA=+Y  FollAlignAxisB=+Y  BaseAlignAxisB=+Z  RotationMatrix=[1 0 0; 0 1 0; 0 0 1]  BlockFunction=simmechanics.library.frames_transforms.rigid_transform
  Transform6 : sm_lib/Frames and Transforms/Rigid Transform  TranslationMethod=Cartesian  TranslationLengthUnit=mm  TranslationStandardAxis=+Z  TranslationStandardOffset=0  TranslationCartesianOffset=[0 -0.59999999999999121 54.041022897086762]  TranslationROffset=0  TranslationROffsetUnits=m  TranslationZOffset=0  TranslationZOffsetUnits=m  TranslationThetaOffset=0  TranslationThetaOffsetUnits=deg  RotationMethod=ArbitraryAxis  RotationAngleUnits=rad  RotationStandardAxis=+Z  RotationAngle=0.37451148767691878  RotationArbitraryAxis=[0 0 1]  FollAlignAxisA=+X  BaseAlignAxisA=+Y  FollAlignAxisB=+Y  BaseAlignAxisB=+Z  RotationMatrix=[1 0 0; 0 1 0; 0 0 1]  BlockFunction=simmechanics.library.frames_transforms.rigid_transform
  Transform7 : sm_lib/Frames and Transforms/Rigid Transform  TranslationMethod=Cartesian  TranslationLengthUnit=mm  TranslationStandardAxis=+Z  TranslationStandardOffset=0  TranslationCartesianOffset=[11.349999999999964 24.800000000000008 98.900000000000077]  TranslationROffset=0  TranslationROffsetUnits=m  TranslationZOffset=0  TranslationZOffsetUnits=m  TranslationThetaOffset=0  TranslationThetaOffsetUnits=deg  RotationMethod=ArbitraryAxis  RotationAngleUnits=rad  RotationStandardAxis=+Z  RotationAngle=1.6887400675970146  RotationArbitraryAxis=[0.32447174056373984 0.8885022111120906 -0.32447174056374006]  FollAlignAxisA=+X  BaseAlignAxisA=+Y  FollAlignAxisB=+Y  BaseAlignAxisB=+Z  RotationMatrix=[1 0 0; 0 1 0; 0 0 1]  BlockFunction=simmechanics.library.frames_transforms.rigid_transform
  Transform8 : sm_lib/Frames and Transforms/Rigid Transform  TranslationMethod=Cartesian  TranslationLengthUnit=mm  TranslationStandardAxis=+Z  TranslationStandardOffset=0  TranslationCartesianOffset=[11.349999999999993 -11.200000000000015 98.900000000000063]  TranslationROffset=0  TranslationROffsetUnits=m  TranslationZOffset=0  TranslationZOffsetUnits=m  TranslationThetaOffset=0  TranslationThetaOffsetUnits=deg  RotationMethod=ArbitraryAxis  RotationAngleUnits=rad  RotationStandardAxis=+Z  RotationAngle=1.9089749650914738  RotationArbitraryAxis=[-0.49911850146428077 0.70835121443539706 0.49911850146428055]  FollAlignAxisA=+X  BaseAlignAxisA=+Y  FollAlignAxisB=+Y  BaseAlignAxisB=+Z  RotationMatrix=[1 0 0; 0 1 0; 0 0 1]  BlockFunction=simmechanics.library.frames_transforms.rigid_transform
  Transform9 : sm_lib/Frames and Transforms/Rigid Transform  TranslationMethod=Cartesian  TranslationLengthUnit=mm  TranslationStandardAxis=+Z  TranslationStandardOffset=0  TranslationCartesianOffset=[0 -14.200000000000031 98.900000000000063]  TranslationROffset=0  TranslationROffsetUnits=m  TranslationZOffset=0  TranslationZOffsetUnits=m  TranslationThetaOffset=0  TranslationThetaOffsetUnits=deg  RotationMethod=ArbitraryAxis  RotationAngleUnits=rad  RotationStandardAxis=+Z  RotationAngle=1.5745392371277764  RotationArbitraryAxis=[0.061065084305083651 0.99626407691817642 -0.06106508430508386]  FollAlignAxisA=+X  BaseAlignAxisA=+Y  FollAlignAxisB=+Y  BaseAlignAxisB=+Z  RotationMatrix=[1 0 0; 0 1 0; 0 0 1]  BlockFunction=simmechanics.library.frames_transforms.rigid_transform
  F1 : PMIOPort  Port=1  Side=Left
  F : PMIOPort  Port=2  Side=Right
  connections:
  Rotor_moteur_roulis_1_RIGID/RConn1 -- ReferenceFrame/RConn1 -- Transform/LConn1 -- Transform1/LConn1 -- Transform10/LConn1 -- Transform11/LConn1 -- Transform12/LConn1 -- Transform13/LConn1 -- Transform14/LConn1 -- Transform15/LConn1 -- Transform16/LConn1 -- Transform17/LConn1 -- Transform18/LConn1 -- Transform19/LConn1 -- Transform2/LConn1 -- Transform8/LConn1 -- Transform9/LConn1 -- Transform7/LConn1 -- Transform6/LConn1 -- Transform5/LConn1 -- Transform4/LConn1 -- Transform3/LConn1 -- Transform27/LConn1 -- Transform26/LConn1 -- Transform25/LConn1 -- Transform24/LConn1 -- Transform23/LConn1 -- Transform22/LConn1 -- Transform21/LConn1 -- Transform20/LConn1
  Transform/RConn1 -- F/RConn1
  STD_M700004_PZ99_KA22x8_KA22_x_8_3_RIGID/LConn1 -- Transform9/RConn1
  STD_M700004_PZ99_KA22x8_KA22_x_8_4_RIGID/LConn1 -- Transform10/RConn1
  STD_M700002_P_KA22x14_1_RIGID/LConn1 -- Transform11/RConn1
  STD_M700004_PZ99_KA22x8_KA22_x_8_5_RIGID/LConn1 -- Transform12/RConn1
  STD_M700004_PZ99_KA22x8_KA22_x_8_6_RIGID/LConn1 -- Transform13/RConn1
  STD_M700002_P_KA22x14_2_RIGID/LConn1 -- Transform14/RConn1
  STD_M700004_PZ99_KA22x8_KA22_x_8_7_RIGID/LConn1 -- Transform15/RConn1
  STD_M700004_PZ99_KA22x8_KA22_x_8_8_RIGID/LConn1 -- Transform16/RConn1
  ALD_M840030_P_Portescap_22NT_82_213P_Z13_Default_1_RIGID/LConn1 -- Transform17/RConn1
  ALD_M100016_P_axe_3x27_3_1_RIGID/LConn1 -- Transform18/RConn1
  Transform1/RConn1 -- F1/RConn1
  ALD_M100015_P_axe_2x13_1_RIGID/LConn1 -- Transform19/RConn1
  STD_M710004_P_vis_M2x5_ALD_M710004_PZ99_vis_M2x5_1_RIGID/LConn1 -- Transform20/RConn1
  STD_M710004_P_vis_M2x5_ALD_M710004_PZ99_vis_M2x5_2_RIGID/LConn1 -- Transform21/RConn1
  STD_M710004_P_vis_M2x5_ALD_M710004_PZ99_vis_M2x5_3_RIGID/LConn1 -- Transform22/RConn1
  ALD_M100004_P_axe_Y_B00_1_RIGID/LConn1 -- Transform23/RConn1
  STD_M510004_P_palier_GFM_1517_05_stabdard_1_RIGID/LConn1 -- Transform24/RConn1
  STD_M510004_P_palier_GFM_1517_05_stabdard_2_RIGID/LConn1 -- Transform25/RConn1
  ALD_M010016_P_roue_sortie_inf_1_RIGID/LConn1 -- Transform26/RConn1
  ALD_M010053_P_support_aimant_1_RIGID/LConn1 -- Transform27/RConn1
  ALD_M010035_P_couvercle_X_AR_Axx_1_RIGID/LConn1 -- Transform2/RConn1
  ALD_M010030_P_cage_fut_moteur_cheville_gauche_Axx_1_RIGID/LConn1 -- Transform3/RConn1
  ALD_M010033_P_couvercle_X_AV_cheville_A02_1_RIGID/LConn1 -- Transform4/RConn1
  ALD_M010055_P_cache_fut_moteur_cheville_A_1_RIGID/LConn1 -- Transform5/RConn1
  ALD_M010292_P_Motor_Ring_Default_1_RIGID/LConn1 -- Transform6/RConn1
  STD_M700004_PZ99_KA22x8_KA22_x_8_1_RIGID/LConn1 -- Transform7/RConn1
  STD_M700004_PZ99_KA22x8_KA22_x_8_2_RIGID/LConn1 -- Transform8/RConn1
